simulink model "windEmulatorStep4"  (R2025b)
settings: Solver=ode4  StartTime=0.0  StopTime=inf  FixedStep=Ts  RelTol=1e-3
values from neighbouring files (symbols this model uses):
  A = 1.0    (= 1)    [initStep4.m]
  absEncoderCountsToRad = 1/2^20*2*pi    (= 5.99211245268e-06)    [initStep4.m]
  acs800CtrlStruct =     [windEmulatorBusDefs.mat]
  acs800DcBusVoltsScaling = 1    [initStep4.m]
  acs800FreqScaling = 1/100    (= 0.01)    [initStep4.m]
  acs800PowerScaling = Gen_PowerScaling    (= 14.9109)    [initStep4.m]
  acs800SignalStruct =     [windEmulatorBusDefs.mat]
  acs800SpeedNomEng = 1500    [initStep4.m]
  acs800SpeedNomFb = 20000    [initStep4.m]
  acs800SpeedScaling = 1500/20000    (= 0.075)    [initStep4.m]
  acs800TempScaling = 1/10    (= 0.1)    [initStep4.m]
  acs800TorqueNomEng = 100    [initStep4.m]
  acs800TorqueNomFb = 10000    [initStep4.m]
  acs800TorqueScaling = acs800TorqueRating/10000    (= 0.008035933)    [initStep4.m]
  acs880CtrlStruct =     [windEmulatorBusDefs.mat]
  acs880FreqScaling = 60/20000    (= 0.003)    [initStep4.m]
  acs880MotorCurrentScaling = 100/10000    (= 0.01)    [initStep4.m]
  acs880MotorVoltsScaling = 1    [initStep4.m]
  acs880PowerScaling = 100*hp2W/10000    (= 7.457)    [initStep4.m]
  acs880RatedTorque = 80.494    [initStep4.m]
  acs880RateLimFalling = -10000    [initStep4.m]
  acs880RateLimRising = 10000    [initStep4.m]
  acs880SetpointLimLower = -0.975*acs880RatedTorque    (= -78.48165)    [initStep4.m]
  acs880SetpointLimUpper = 0.975*acs880RatedTorque    (= 78.48165)    [initStep4.m]
  acs880SignalStruct =     [windEmulatorBusDefs.mat]
  acs880SpeedPILimLo = -0.975*acs880RatedTorque    (= -78.48165)    [initStep4.m]
  acs880SpeedPILimUp = 0.975*acs880RatedTorque    (= 78.48165)    [initStep4.m]
  acs880SpeedScaling = 2000/20000    (= 0.1)    [initStep4.m]
  acs880TorqueFieldbusScale = 10000    [initStep4.m]
  acs880TorqueScaling = acs880RatedTorque/acs880TorqueFieldbusScale    (= 0.0080494)    [initStep4.m]
  acs880TorqueSetpointScaling = 100    [initStep4.m]
  bar2pa = 1e5    (= 100000)    [initStep4.m]
  belowMinPGain = 1/200    (= 0.005)    [initStep4.m]
  ctrlModeTorque = logical(true)    [init.m]    (also in initStep1.m; initStep2.m; initStep3.m; initStep4.m)
  ctrlSignal1 = squeeze(hptoSignalsData.Values.ctrlSignal1.Data)    [postProcessingStep2.m]
  ctrlSignal2 = squeeze(hptoSignalsData.Values.ctrlSignal2.Data)    [postProcessingStep2.m]
  deadBandController = boolean(false)    [initStep4.m]
  deadbandTorqueSlewRate = 300    [initStep4.m]
  Dm_max = 40    [initStep4.m]
  EffMechMax = 0.93    [initStep4.m]
  EffMechMin = 0.79    [initStep4.m]
  excForce_N = squeeze(hptoCtrlData.Values.excForce_N.Data)    [postProcessingStep2.m]
  expCtrlStruct =     [windEmulatorBusDefs.mat]
  FactorEff = psi2pa*cc2m3*(1/rev2rad)    (= 0.00109733470463)    [initStep4.m]
  fromFileSpeedSlewRate = 250    [initStep4.m]
  fromFileTorqueSlewRate = 25    [initStep4.m]
  futekTorqueScale = -1/(2^31)*10/5*100    (= -9.31322574615e-08)    [initStep4.m]
  genMaxTorque = 0.8*ratedTorque    (= 64.3952)    [initStep3.m]    (also in initStep4.m = 78.48165)
  genTorqueCmd_Nm = squeeze(hptoSignalsData.Values.genTorqueCmd_Nm.Data)    [postProcessingStep2.m]
  hbmCtScale = 1/1.5    (= 0.666666666667)    [initStep4.m]
  hbmPowerStruct =     [windEmulatorBusDefs.mat]
  hptoCtrlStruct =     [windEmulatorBusDefs.mat]
  hptoSignalStruct =     [windEmulatorBusDefs.mat]
  invPowerStruct =     [windEmulatorBusDefs.mat]
  lpm2m3ps = 1/m3ps2lpm    (= 1.66666666667e-05)    [initStep4.m]
  minPressureRef_psi = 1000    [initStep4.m]
  minTorqueRef_Nm = (minPressureRef_psi*psi2pa)*(Dm_max*cc2m3*(1/rev2rad))    (= 43.8933881851)    [initStep4.m]
  motorSpeed_rpm = squeeze(acs880SignalsData.Values.motorSpeed_rpm.Data)    [postProcessingStep2.m]
  nPreDrop = 2900    [initStep4.m]
  nPreDropMin = 725    [initStep4.m]
  psi2bar = 1/bar2psi    (= 0.0689475729318)    [initStep4.m]
  radps2rpm = 60/(2*pi)    (= 9.54929658551)    [initStep2.m]    (also in initStep4.m)
  rpm2radps = 2*pi/60    (= 0.10471975512)    [initStep4.m]
  runCounter = squeeze(hptoCtrlData.Values.runCounter.Data)    [postProcessingStep2.m]
  shaftSignalStruct =     [windEmulatorBusDefs.mat]
  sidCtrlStruct =     [windEmulatorBusDefs.mat]
  sidDataCaseCounter = sidData.experimentData.count    [initStep4.m]
  sidDataSpeed_rpm = sidData.experimentData.wShaft_rpm    [initStep4.m]
  sidDataTorque_Nm = sidData.experimentData.torqueShaft_Nm    [initStep4.m]
  sidInfoStruct =     [windEmulatorBusDefs.mat]
  T = 4    [initStep4.m]
  targetOmega = 2000/60*2*pi    (= 209.439510239)    [initStep2.m]    (also in initStep3.m; initStep4.m)
  time = hptoCtrlData.Values.runCounter.Time    [postProcessingStep2.m]
  TorqueLoadMax = 75    [initStep4.m]
  Ts = 1/250    (= 0.004)    [initStep4.m]
undefined symbols (not defined in the file or in its folder): absEncoderCounts, absEncoderPosition_rad, absEncoderSpeed_rpm, absEncoderStatus1, absEncoderStatus2, absEncoderTurns, acs800Torque_Nm, acs800TorqueSetpoint_Nm, acs880SpeedSetpoint_rpm, acs880Torque_Nm, ctrlWord, dcBusVoltage_V, DiscIntNeverNeededParam, excShaftSpeed_rpm, excShaftTorque_Nm, expType, expTypeEnum, frequency_Hz, fromFileCaseCounter, genPumpFlow_lpm, genShaftSpeed_rpm, genSpeedActual, hmOutputShafTorque_Nm, motorCurrent_A, motorTorque_Nm, motorVoltage_V, pressure_bar, PressureControl, ramp, resetHilIntegrator, resetSidIntegrator, runHil, runSid, shaftPower_W, sidType, sidTypeEnum, SpeedControl, speedCtrlReset, speedRef_rpm, state, statusWord, stepCounter, temperature, torqueActual_Nm, TorqueInputControl, torqueSetpoint_Nm, torqueSetpoint_percent
libraries: slrealtimeethercatlib x118, fl_lib x26, nesl_utility x17, slrealtimeloglib x13, sh_lib x9, dspstat3 x5, simulink_extras x4, slpidlib x3, cstblocks x3, dspindex x3, simulink x2
(part 1 of 5)
settings Model: SimulationMode=external  Creator=SWEPT  LastModifiedBy=jleonqu
settings SolverCC: ConcurrentTasks=on  PositivePriorityOrder=on
settings DataIOCC: ExternalInput=inputData  LoadExternalInput=on
settings OptimizationCC: BlockReduction=off  OptimizeBlockIOStorage=off  ReuseModelBlockBuffer=off
settings DebuggingCC: TasksWithSamePriorityMsg=none  UnconnectedInputMsg=warning  UnconnectedOutputMsg=warning  UnconnectedLineMsg=warning
settings HardwareCC: ProdBitPerLong=64.0  ProdLongLongMode=on  ProdHWDeviceType=Intel->x86-64 (Linux 64)
settings ModelReferenceCC: EnableRefExpFcnMdlSchedulingChecks=on
settings RTWCC: SystemTargetFile=speedgoat.tlc  TemplateMakefile=slrealtime_default_tmf  RTWVerbose=off  Toolchain=Simulink Real-Time Toolchain  BuildConfiguration=Faster Runs  CodeExecutionProfiling=on  TargetLang=C++  GPUComputeCapability=3.5  DLArmComputeVersion=19.05  Description=Speedgoat Real-Time Target Machine
settings SimulinkRealTimeTargetCC: SLRTFileLogMaxRuns=1.0  ExtModeMaxTrigDuration=10.0  ExtModeStaticAllocSize=1000000.0  ExtModeTransport=0.0  MultiwordLength=2048.0  DynamicStringBufferSize=256.0  PreserveMATLABNamespacesInGeneratedCode=on  SubcomponentCodeInterfacePackaging=Reusable function  MATLABClassNameForMDSCustomization=Simulink.SoftwareTarget.GRTCustomization  InstructionSetFMA=off  LogToMDFFile=off

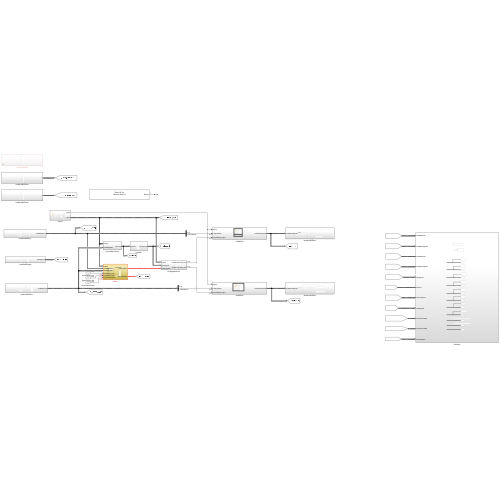
[thumbnail: Simulink's stored preview of the top-level diagram]
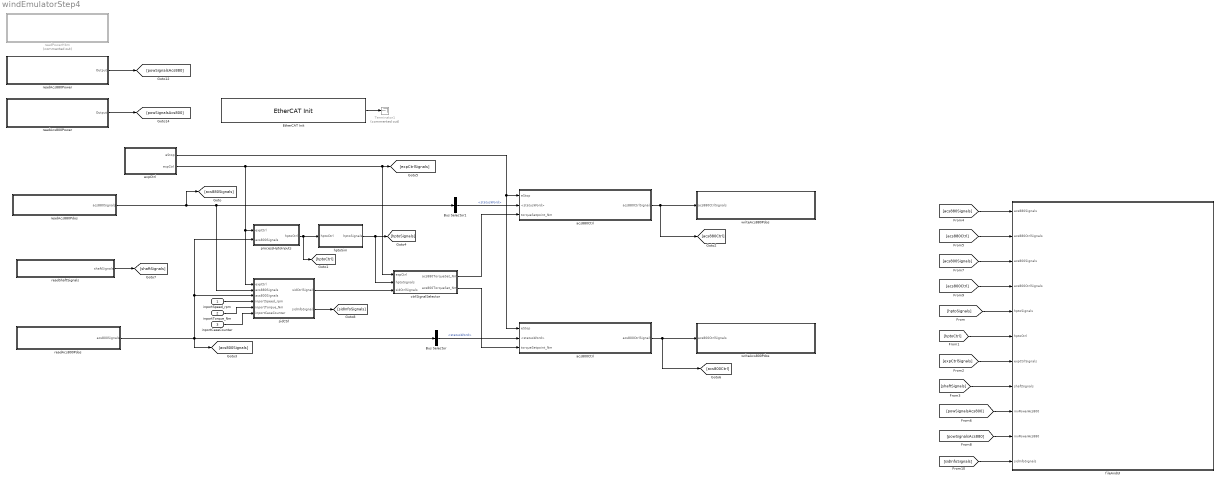
== system windEmulatorStep4 ==
  inportSpeed_rpm : Inport  Interpolate=off
  inportTorque_Nm : Inport  Port=2  Interpolate=off
  inportCaseCounter : Inport  Port=3  Interpolate=off
  Bus Selector : BusSelector  OutputSignals=statusWord
  Bus Selector1 : BusSelector  OutputSignals=statusWord
  EtherCAT Init : slrealtimeethercatlib/EtherCAT Init  Priority=0  config_file=C:\Users\jleonqu\Documents\GitHub\WEC-Sim_Applications\WEC-Sim_HIL\WindEmulatorFiles_edited\ethercat\newDevice3File_windEmulator_noHBM-2026-06-26.xml  device_id=0  portnum=1  initstate=2  dctuning=2  enaDebug=1  logFile='c:\dbglog.txt'  sample_time=0.004000  DCMode=0
  Terminator1 : Terminator  Commented=on
  acs800Ctrl : Subsystem
  acs880Ctrl : Subsystem
  ctrlSignalSelector : Subsystem
  expCtrl : Subsystem
  fileAndUI : Subsystem
  hptoSim : Subsystem
  processHptoInputs : Subsystem
  readAcs800Pdos : Subsystem
  readAcs800Power : Subsystem
  readAcs880Pdos : Subsystem
  readAcs880Power : Subsystem
  readPowerHbm : Subsystem  Commented=on
  readShaftSignals : Subsystem
  sidCtrl : Subsystem
  writeAcs800Pdos : Subsystem
  writeAcs880Pdos : Subsystem
  wires:
  EtherCAT Init/1 -> Terminator1/1
  readAcs800Pdos/1(acs800Signals) -> Bus Selector/1, [acs800Signals], processHptoInputs/2(acs800Signals), sidCtrl/3(acs800Signals)
  readAcs880Pdos/1(acs880Signals) -> sidCtrl/2(acs880Signals), Bus Selector1/1, [acs880Signals]
  Bus Selector1/1 -> acs880Ctrl/2(<statusWord>)  "<statusWord>"
  acs880Ctrl/1(acs880CtrlSignals) -> [acs880Ctrl], writeAcs880Pdos/1(acs880CtrlSignals)
  [acs880Signals] -> fileAndUI/1(acs880Signals)
  [acs880Ctrl] -> fileAndUI/2(acs880CtrlSignals)
  Bus Selector/1 -> acs800Ctrl/2(<statusWord>)  "<statusWord>"
  hptoSim/1(hptoSignals) -> ctrlSignalSelector/2(hptoSignals), [hptoSignals]
  expCtrl/1(eStop) -> acs800Ctrl/1(eStop), acs880Ctrl/1(eStop)
  acs800Ctrl/1(acs800CtrlSignals) -> [acs800Ctrl], writeAcs800Pdos/1(acs800CtrlSignals)
  [acs800Signals] -> fileAndUI/3(acs800Signals)
  [acs800Ctrl] -> fileAndUI/4(acs800CtrlSignals)
  processHptoInputs/1(hptoCtrl) -> [hptoCtrl], hptoSim/1(hptoCtrl)
  [hptoSignals] -> fileAndUI/5(hptoSignals)
  [hptoCtrl] -> fileAndUI/6(hptoCtrl)
  sidCtrl/1(sidCtrlSignals) -> ctrlSignalSelector/3(sidCtrlSignals)
  ctrlSignalSelector/1(acs880TorqueSet_Nm) -> acs880Ctrl/3(torqueSetpoint_Nm)
  ctrlSignalSelector/2(acs800TorqueSet_Nm) -> acs800Ctrl/3(torqueSetpoint_Nm)
  [expCtrlSignals] -> fileAndUI/7(expCtrlSignals)
  readShaftSignals/1(shaftSignals) -> [shaftSignals]
  [shaftSignals] -> fileAndUI/8(shaftSignals)
  expCtrl/2(expCtrl) -> ctrlSignalSelector/1(expCtrl), [expCtrlSignals], sidCtrl/1(expCtrl), processHptoInputs/1(expCtrl)
  readAcs800Power/1(Output) -> [powSignalsAcs800]
  readAcs880Power/1(Output) -> [powSignalsAcs880]
  [powSignalsAcs800] -> fileAndUI/9(invPowerAcs800)
  [powSignalsAcs880] -> fileAndUI/10(invPowerAcs880)
  sidCtrl/2(sidInfoSignals) -> [sidInfoSignals]
  [sidInfoSignals] -> fileAndUI/11(sidInfoSignals)
  inportSpeed_rpm/1 -> sidCtrl/4(inportSpeed_rpm)
  inportTorque_Nm/1 -> sidCtrl/5(inportTorque_Nm)
  inportCaseCounter/1 -> sidCtrl/6(inportCaseCounter)

== system windEmulatorStep4/acs800Ctrl ==
  note: Any limiting of the torque setpoint here?
  note: ideally change this; needs change to ctrlWord type
  note: ACS800 state control
  note: Act on change of button
  eStop : Inport  OutDataTypeStr=boolean
  <statusWord> : Inport  Port=2
  torqueSetpoint_Nm : Inport  Port=3
  ACS800CtrlMode : Constant  Value=ctrlModeTorque  OutDataTypeStr=boolean
  ACS880FieldbusControl : Subsystem
  Bus Assignment : BusAssignment  AssignedSignals=ctrlWord,state,torqueSetpoint_Nm,torqueSetpoint_percent
  Cast To Double : DataTypeConversion  OutDataTypeStr=double  SaturateOnIntegerOverflow=off  RndMeth=Floor
  Cast To Double1 : DataTypeConversion  OutDataTypeStr=int32  SaturateOnIntegerOverflow=off  RndMeth=Floor
  Constant : Constant  Value=acs800CtrlStruct  OutDataTypeStr=Bus: acs800CtrlBus
  Memory : Memory
  Memory1 : Memory
  Memory2 : Memory
  "Nm -> %" : Gain  Gain=1/acs880RatedTorque*100
  NotEqual : RelationalOperator  Operator=~=  OutDataTypeStr=boolean  RndMeth=Simplest  InputSameDT=off
  NotEqual1 : RelationalOperator  Operator=~=  OutDataTypeStr=boolean  RndMeth=Simplest  InputSameDT=off
  NotEqual2 : RelationalOperator  Operator=~=  OutDataTypeStr=boolean  RndMeth=Simplest  InputSameDT=off
  powerDownButton : Constant  Value=false
  powerUpButton : Constant  Value=false
  resetFaultButton : Constant  Value=false
  acs800CtrlSignals : Outport  OutDataTypeStr=Bus: acs800CtrlBus
  wires:
  <statusWord>/1 -> ACS880FieldbusControl/5(StatusWord)
  powerUpButton/1 -> NotEqual/1, Memory/1
  Memory/1 -> NotEqual/2
  ACS800CtrlMode/1 -> ACS880FieldbusControl/6(ctrlMode)
  Memory1/1 -> NotEqual1/2
  powerDownButton/1 -> NotEqual1/1, Memory1/1
  resetFaultButton/1 -> Memory2/1, NotEqual2/1
  Memory2/1 -> NotEqual2/2
  NotEqual/1 -> ACS880FieldbusControl/1(powerUp)
  NotEqual1/1 -> ACS880FieldbusControl/2(powerDown)
  eStop/1 -> ACS880FieldbusControl/4(eStop)
  ACS880FieldbusControl/2(state) -> Cast To Double1/1
  NotEqual2/1 -> Cast To Double/1
  Cast To Double/1 -> ACS880FieldbusControl/3(resetFault)
  Constant/1 -> Bus Assignment/1
  ACS880FieldbusControl/1(ControlWord) -> Bus Assignment/2
  Bus Assignment/1 -> acs800CtrlSignals/1
  Cast To Double1/1 -> Bus Assignment/3
  torqueSetpoint_Nm/1 -> Bus Assignment/4, "Nm -> %"/1
  "Nm -> %"/1 -> Bus Assignment/5

== system windEmulatorStep4/acs880Ctrl ==
  note: ideally change this; needs change to ctrlWord type
  note: ACS880 Control Word
  note: Act on change of button
  note: Should not need this ramp anymore; this was originally used for manual (constant) torque setpoints
  note: ACS880 Torque setpoint limit and conversion
  eStop : Inport  OutDataTypeStr=boolean
  <statusWord> : Inport  Port=2
  torqueSetpoint_Nm : Inport  Port=3  OutDataTypeStr=double
  ACS880CtrlMode : Constant  Value=ctrlModeTorque  OutDataTypeStr=boolean
  ACS880FieldbusControl : Subsystem
  ACS880Ramp : Stateflow chart  Commented=on  TreatAsAtomicUnit=on
  ACS880Setpoint : Product  Commented=on
  Bus Assignment : BusAssignment  AssignedSignals=ctrlWord,state,torqueSetpoint_Nm,torqueSetpoint_percent
  Cast To Double : DataTypeConversion  OutDataTypeStr=double  SaturateOnIntegerOverflow=off  RndMeth=Floor
  Cast To Double1 : DataTypeConversion  OutDataTypeStr=int32  SaturateOnIntegerOverflow=off  RndMeth=Floor
  Constant : Constant  Value=acs880CtrlStruct  OutDataTypeStr=Bus: acs880CtrlBus
  Memory : Memory
  Memory1 : Memory
  Memory2 : Memory
  "Nm -> %" : Gain  Gain=1/acs880RatedTorque*100
  NotEqual : RelationalOperator  Operator=~=  OutDataTypeStr=boolean  RndMeth=Simplest  InputSameDT=off
  NotEqual1 : RelationalOperator  Operator=~=  OutDataTypeStr=boolean  RndMeth=Simplest  InputSameDT=off
  NotEqual2 : RelationalOperator  Operator=~=  OutDataTypeStr=boolean  RndMeth=Simplest  InputSameDT=off
  Saturation : Saturate  UpperLimit=acs880SetpointLimUpper  LowerLimit=acs880SetpointLimLower
  acs880RateLim : RateLimiter  RisingSlewLimit=acs880RateLimRising  FallingSlewLimit=acs880RateLimFalling  SampleTimeMode=inherited
  powerDownButton : Constant  Value=false
  powerUpButton : Constant  Value=false
  resetFaultButton : Constant  Value=false
  acs880CtrlSignals : Outport  OutDataTypeStr=Bus: acs880CtrlBus
  wires:
  <statusWord>/1 -> ACS880FieldbusControl/5(StatusWord)
  powerUpButton/1 -> NotEqual/1, Memory/1
  Memory/1 -> NotEqual/2
  ACS880CtrlMode/1 -> ACS880FieldbusControl/6(ctrlMode)
  Memory1/1 -> NotEqual1/2
  powerDownButton/1 -> NotEqual1/1, Memory1/1
  resetFaultButton/1 -> Memory2/1, NotEqual2/1
  Memory2/1 -> NotEqual2/2
  NotEqual/1 -> ACS880FieldbusControl/1(powerUp)
  NotEqual1/1 -> ACS880FieldbusControl/2(powerDown)
  eStop/1 -> ACS880FieldbusControl/4(eStop)
  ACS880FieldbusControl/2(state) -> Cast To Double1/1
  NotEqual2/1 -> Cast To Double/1
  Cast To Double/1 -> ACS880FieldbusControl/3(resetFault)
  Constant/1 -> Bus Assignment/1
  ACS880FieldbusControl/1(ControlWord) -> Bus Assignment/2
  Bus Assignment/1 -> acs880CtrlSignals/1
  Cast To Double1/1 -> Bus Assignment/3
  ACS880Ramp/1(ramp) -> ACS880Setpoint/2  "rampValue"
  acs880RateLim/1 -> Saturation/1
  Saturation/1 -> "Nm -> %"/1, Bus Assignment/4  "ACS880Setpoint"
  torqueSetpoint_Nm/1 -> acs880RateLim/1
  "Nm -> %"/1 -> Bus Assignment/5

== system windEmulatorStep4/ctrlSignalSelector ==
  note: Modes:
      |
      | Off
      | Torque setpoint to both drives zero.
      |
      | SID
      | Torque setpoint to both drives taken from SID control signals.
      |
      | HIL
      | ACS880: simulates hydraulic machine (HM) output shaft
      | ACS800: provides the generator torque
  expCtrl : Inport  OutDataTypeStr=Bus: expCtrlBus
  hptoSignals : Inport  Port=2  OutDataTypeStr=Bus: hptoSignalBus
  sidCtrlSignals : Inport  Port=3  OutDataTypeStr=Bus: sidCtrlBus
  Bus Selector : BusSelector  OutputSignals=hmOutputShafTorque_Nm,genTorqueCmd_Nm
  Bus Selector1 : BusSelector  OutputSignals=acs880Torque_Nm,acs800Torque_Nm
  Bus Selector2 : BusSelector  OutputSignals=expType
  Multiport Switch : MultiPortSwitch  DataPortOrder=Specify indices  DataPortIndices={expTypeEnum.off,expTypeEnum.sid,expTypeEnum.hil}  DataPortForDefault=Additional data port  SaturateOnIntegerOverflow=off  InputSameDT=off
  Multiport Switch1 : MultiPortSwitch  DataPortOrder=Specify indices  DataPortIndices={expTypeEnum.off,expTypeEnum.sid,expTypeEnum.hil}  DataPortForDefault=Additional data port  SaturateOnIntegerOverflow=off  InputSameDT=off
  toExpTypeEnum : DataTypeConversion  OutDataTypeStr=Enum: expTypeEnum  SaturateOnIntegerOverflow=off  RndMeth=Floor
  zeroTorque : Constant  Value=0  OutDataTypeStr=double
  acs880TorqueSet_Nm : Outport
  acs800TorqueSet_Nm : Outport  Port=2
  wires:
  hptoSignals/1 -> Bus Selector/1
  sidCtrlSignals/1 -> Bus Selector1/1
  Multiport Switch/1 -> acs880TorqueSet_Nm/1
  Multiport Switch1/1 -> acs800TorqueSet_Nm/1
  zeroTorque/1 -> Multiport Switch1/5, Multiport Switch1/2, Multiport Switch/5, Multiport Switch/2
  Bus Selector1/1 -> Multiport Switch/3  "<acs880Torque_Nm>"
  Bus Selector1/2 -> Multiport Switch1/3  "<acs800Torque_Nm>"
  Bus Selector/1 -> Multiport Switch/4  "<hmOutputShafTorque_Nm>"
  Bus Selector/2 -> Multiport Switch1/4  "<genTorqueCmd_Nm>"
  Bus Selector2/1 -> toExpTypeEnum/1  "<expType>"
  expCtrl/1 -> Bus Selector2/1
  toExpTypeEnum/1 -> Multiport Switch1/1, Multiport Switch/1

== system windEmulatorStep4/expCtrl ==
  note: Act on change of button
  note: Act on change of button
  note: Act on change of button
  Bus Assignment : BusAssignment  AssignedSignals=expType,runHil,runSid,time,ramp,runCounter,stepCounter,resetHilIntegrator,resetSidIntegrator
  Constant : Constant  Value=expCtrlStruct  OutDataTypeStr=Bus: expCtrlBus
  Equal : RelationalOperator  Operator===  OutDataTypeStr=boolean  RndMeth=Simplest  InputSameDT=off
  Equal1 : RelationalOperator  Operator===  OutDataTypeStr=boolean  RndMeth=Simplest  InputSameDT=off
  FexcRamp : Stateflow chart  TreatAsAtomicUnit=on
  Memory : Memory
  Memory1 : Memory
  Memory2 : Memory
  NotEqual : RelationalOperator  Operator=~=  OutDataTypeStr=boolean  RndMeth=Simplest  InputSameDT=off
  NotEqual1 : RelationalOperator  Operator=~=  OutDataTypeStr=boolean  RndMeth=Simplest  InputSameDT=off
  NotEqual2 : RelationalOperator  Operator=~=  OutDataTypeStr=boolean  RndMeth=Simplest  InputSameDT=off
  ToUint16 : DataTypeConversion  OutDataTypeStr=uint16  SaturateOnIntegerOverflow=off  RndMeth=Floor
  eStopButton : Constant  Value=false
  expModeHil : Constant  Value=expTypeEnum.hil  OutDataTypeStr=Enum: expTypeEnum
  expModeSid : Constant  Value=expTypeEnum.sid  OutDataTypeStr=Enum: expTypeEnum
  expRunTime : Constant  Value=0
  expType : Constant  Value=expTypeEnum.off  OutDataTypeStr=Enum: expTypeEnum
  startButton : Constant  Value=false
  stopButton : Constant  Value=false
  eStop : Outport
  expCtrl : Outport  Port=2  OutDataTypeStr=Bus: expCtrlBus
  wires:
  eStopButton/1 -> NotEqual/1, Memory/1
  NotEqual/1 -> eStop/1
  Memory/1 -> NotEqual/2
  Bus Assignment/1 -> expCtrl/1
  Constant/1 -> Bus Assignment/1
  ToUint16/1 -> Bus Assignment/2
  expType/1 -> FexcRamp/1(expType), Equal1/1, Equal/1, ToUint16/1
  Memory1/1 -> NotEqual1/2
  startButton/1 -> Memory1/1, NotEqual1/1
  Memory2/1 -> NotEqual2/2
  stopButton/1 -> Memory2/1, NotEqual2/1
  NotEqual1/1 -> FexcRamp/2(startButton)
  NotEqual2/1 -> FexcRamp/3(stopButton)
  expRunTime/1 -> FexcRamp/4(expRunTime)
  FexcRamp/1(time) -> Bus Assignment/5
  FexcRamp/2(ramp) -> Bus Assignment/6  "rampValue"
  FexcRamp/3(runCounter) -> Bus Assignment/7
  Equal/1 -> Bus Assignment/3
  expModeHil/1 -> Equal/2
  Equal1/1 -> Bus Assignment/4
  expModeSid/1 -> Equal1/2
  FexcRamp/5(resetHilIntegrator) -> Bus Assignment/9
  FexcRamp/6(resetSidIntegrator) -> Bus Assignment/10
  FexcRamp/4(stepCounter) -> Bus Assignment/8

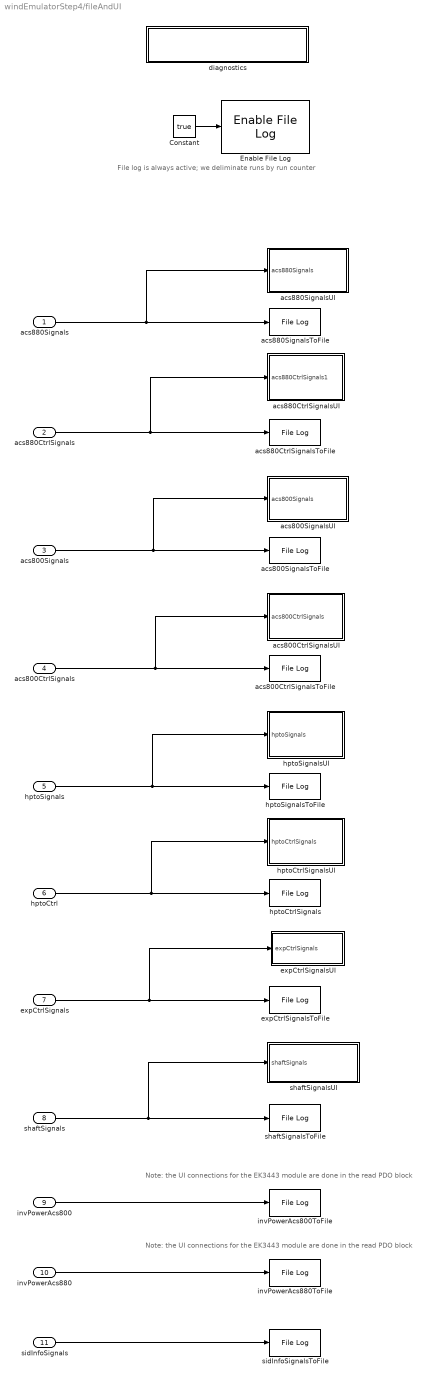
== system windEmulatorStep4/fileAndUI ==
  note: Note: the UI connections for the EK3443 module are done in the read PDO block
  note: File log is always active; we deliminate runs by run counter
  note: Note: the UI connections for the EK3443 module are done in the read PDO block
  acs880Signals : Inport  OutDataTypeStr=Bus: acs880SignalBus
  acs880CtrlSignals : Inport  Port=2  OutDataTypeStr=Bus: acs880CtrlBus
  acs800Signals : Inport  Port=3  OutDataTypeStr=Bus: acs800SignalBus
  acs800CtrlSignals : Inport  Port=4  OutDataTypeStr=Bus: acs800CtrlBus
  hptoSignals : Inport  Port=5  OutDataTypeStr=Bus: hptoSignalBus
  hptoCtrl : Inport  Port=6  OutDataTypeStr=Bus: hptoCtrlBus
  expCtrlSignals : Inport  Port=7  OutDataTypeStr=Bus: expCtrlBus
  shaftSignals : Inport  Port=8  OutDataTypeStr=Bus: shaftSignalBus
  invPowerAcs800 : Inport  Port=9  OutDataTypeStr=Bus: invPowerBus
  invPowerAcs880 : Inport  Port=10  OutDataTypeStr=Bus: invPowerBus
  sidInfoSignals : Inport  Port=11  OutDataTypeStr=Bus: sidInfoBus
  Constant : Constant  Value=true  OutDataTypeStr=boolean
  Enable File Log : slrealtimeloglib/Enable File Log
  acs800CtrlSignalsToFile : slrealtimeloglib/File Log  decimation=fileDecimation  inputProcessing=Elements as channels (sample based)
  acs800CtrlSignalsUI : Subsystem
  acs800SignalsToFile : slrealtimeloglib/File Log  decimation=fileDecimation  inputProcessing=Elements as channels (sample based)
  acs800SignalsUI : Subsystem
  acs880CtrlSignalsToFile : slrealtimeloglib/File Log  decimation=fileDecimation  inputProcessing=Elements as channels (sample based)
  acs880CtrlSignalsUI : Subsystem
  acs880SignalsToFile : slrealtimeloglib/File Log  decimation=fileDecimation  inputProcessing=Elements as channels (sample based)
  acs880SignalsUI : Subsystem
  diagnostics : Subsystem
  expCtrlSignalsToFile : slrealtimeloglib/File Log  decimation=fileDecimation  inputProcessing=Elements as channels (sample based)
  expCtrlSignalsUI : Subsystem
  hptoCtrlSignals : slrealtimeloglib/File Log  decimation=fileDecimation  inputProcessing=Elements as channels (sample based)
  hptoCtrlSignalsUI : Subsystem
  hptoSignalsToFile : slrealtimeloglib/File Log  decimation=fileDecimation  inputProcessing=Elements as channels (sample based)
  hptoSignalsUI : Subsystem
  invPowerAcs800ToFile : slrealtimeloglib/File Log  decimation=fileDecimation  inputProcessing=Elements as channels (sample based)
  invPowerAcs880ToFile : slrealtimeloglib/File Log  decimation=fileDecimation  inputProcessing=Elements as channels (sample based)
  shaftSignalsToFile : slrealtimeloglib/File Log  decimation=fileDecimation  inputProcessing=Elements as channels (sample based)
  shaftSignalsUI : Subsystem
  sidInfoSignalsToFile : slrealtimeloglib/File Log  decimation=fileDecimation  inputProcessing=Elements as channels (sample based)
  wires:
  Constant/1 -> Enable File Log/1
  acs880Signals/1 -> acs880SignalsUI/1(acs880Signals), acs880SignalsToFile/1
  acs880CtrlSignals/1 -> acs880CtrlSignalsUI/1(acs880CtrlSignals1), acs880CtrlSignalsToFile/1
  acs800Signals/1 -> acs800SignalsUI/1(acs800Signals), acs800SignalsToFile/1
  acs800CtrlSignals/1 -> acs800CtrlSignalsUI/1(acs800CtrlSignals), acs800CtrlSignalsToFile/1
  hptoSignals/1 -> hptoSignalsUI/1(hptoSignals), hptoSignalsToFile/1
  hptoCtrl/1 -> hptoCtrlSignalsUI/1(hptoCtrlSignals), hptoCtrlSignals/1
  expCtrlSignals/1 -> expCtrlSignalsUI/1(expCtrlSignals), expCtrlSignalsToFile/1
  shaftSignals/1 -> shaftSignalsToFile/1, shaftSignalsUI/1(shaftSignals)
  invPowerAcs800/1 -> invPowerAcs800ToFile/1
  invPowerAcs880/1 -> invPowerAcs880ToFile/1
  sidInfoSignals/1 -> sidInfoSignalsToFile/1

== system windEmulatorStep4/hptoSim ==
  note: Notes on Step 4:
      |
      | TODO: Review the below text; this is outdated.
      |
      | One drive is in torque control and the other is in speed control.
      |
      | The torque and shaft speed setpoint are produced as the output of the shaft in the hydraulic motor and generator in the hydraulic PTO model.
  hptoCtrl : Inport  OutDataTypeStr=Bus: hptoCtrlBus
  Bus Assignment : BusAssignment  AssignedSignals=genTorqueCmd_Nm,pressure_bar,hmOutputShafTorque_Nm,genShaftSpeed_rpm,excShaftSpeed_rpm,excShaftTorque_Nm,ctrlSignal1,ctrlSignal2,genPumpFlow_lpm
  Bus Selector : BusSelector  OutputSignals=speedRef_rpm,genSpeedActual,excForce_N,speedCtrlReset
  Constant : Constant  Value=hptoSignalStruct  OutDataTypeStr=Bus: hptoSignalBus
  hptoModel : Subsystem
  "psi -> bar" : Gain  Gain=psi2bar
  hptoSignals : Outport  OutDataTypeStr=Bus: hptoSignalBus
  wires:
  hptoModel/9(genPumpFlow_lpm) -> Bus Assignment/10
  hptoModel/3(hmOutputShaftTorque_Nm) -> Bus Assignment/4
  Bus Assignment/1 -> hptoSignals/1
  Constant/1 -> Bus Assignment/1
  hptoModel/4(genShaftSpeed_rpm) -> Bus Assignment/5
  hptoModel/8(controlSignal2) -> Bus Assignment/9
  hptoModel/1(genTorqueCmd_Nm) -> Bus Assignment/2  "genTorque_Nm"
  hptoModel/2(pressure_psi) -> "psi -> bar"/1  "pressure_psi"
  "psi -> bar"/1 -> Bus Assignment/3
  hptoModel/7(controlSignal1) -> Bus Assignment/8
  hptoCtrl/1 -> Bus Selector/1
  Bus Selector/1 -> hptoModel/1(speedReference)  "<speedRef_rpm>"
  Bus Selector/2 -> hptoModel/2(genSpeedActual_rpm)  "<genSpeedActual>"
  Bus Selector/3 -> hptoModel/3(excForce_N)  "<excForce_N>"
  Bus Selector/4 -> hptoModel/4(speedControllerReset)  "<speedCtrlReset>"
  hptoModel/5(excShaftSpeed_rpm) -> Bus Assignment/6
  hptoModel/6(excShaftTorque_Nm) -> Bus Assignment/7

== system windEmulatorStep4/processHptoInputs ==
  note: Keep exciation force at zero if we are not running HIL
  note: This is in (N) for the WaveBot excitation force
  expCtrl : Inport  OutDataTypeStr=Bus: expCtrlBus
  acs800Signals : Inport  Port=2  OutDataTypeStr=Bus: acs800SignalBus
  Bus Assignment : BusAssignment  AssignedSignals=speedRef_rpm,excForce_N,genSpeedActual,speedCtrlReset
  Bus Selector : BusSelector  OutputSignals=ramp,runHil,time,resetHilIntegrator
  Bus Selector2 : BusSelector  OutputSignals=motorSpeed_rpm
  Constant : Constant  Value=hptoCtrlStruct  OutDataTypeStr=Bus: hptoCtrlBus
  Constant1 : Constant  Value=0
  ExcitationForce_N : Product
  Product : Product
  Product4 : Product
  Rate Limiter : RateLimiter  RisingSlewLimit=50  FallingSlewLimit=-50  SampleTimeMode=inherited
  Sin2 : Trigonometry
  Switch : Switch  Criteria=u2 > Threshold  SaturateOnIntegerOverflow=off  InputSameDT=off
  excForceAmpNow_N : Gain
  excForceAmp_N : Constant  Value=0
  excForceFreq_Hz : Constant  Value=0
  f->w : Gain  Gain=2*pi
  speedReference : Constant  Value=0
  hptoCtrl : Outport  OutDataTypeStr=Bus: hptoCtrlBus
  wires:
  speedReference/1 -> Rate Limiter/1
  Rate Limiter/1 -> Bus Assignment/2
  Switch/1 -> Product/2  "rampValue"
  Product4/1 -> Sin2/1
  Sin2/1 -> ExcitationForce_N/1
  acs800Signals/1 -> Bus Selector2/1
  Constant/1 -> Bus Assignment/1
  Bus Assignment/1 -> hptoCtrl/1
  Bus Selector2/1 -> Bus Assignment/4  "<motorSpeed_rpm>"
  excForceFreq_Hz/1 -> f->w/1
  f->w/1 -> Product4/1
  ExcitationForce_N/1 -> Product/1  "waveBotExcitationForce_N"
  Product/1 -> Bus Assignment/3
  excForceAmp_N/1 -> excForceAmpNow_N/1
  excForceAmpNow_N/1 -> ExcitationForce_N/2
  expCtrl/1 -> Bus Selector/1
  Bus Selector/3 -> Product4/2  "<time>"
  Bus Selector/2 -> Switch/2  "<runHil>"
  Bus Selector/1 -> Switch/1  "<ramp>"
  Constant1/1 -> Switch/3
  Bus Selector/4 -> Bus Assignment/5  "<resetHilIntegrator>"

== system windEmulatorStep4/readAcs800Pdos ==
  Bus Assignment : BusAssignment  AssignedSignals=dcBusVoltage_V,frequency_Hz,temperature,motorSpeed_rpm,motorTorque_Nm,shaftPower_W,statusWord
  Constant : Constant  Value=acs800SignalStruct  OutDataTypeStr=Bus: acs800SignalBus
  Data Type Conversion{,1..5} (6 alike) : DataTypeConversion  OutDataTypeStr=double  SaturateOnIntegerOverflow=off  RndMeth=Floor
  EtherCAT PDO Receive10 : slrealtimeethercatlib/EtherCAT PDO Receive  Priority=2  sig_name=ACS800.TxPDO 1.Converter Temperature  sig_offset=632  sig_type=int16  type_size=16  sig_dim=1  device_id=0  sample_time=0.004000
  EtherCAT PDO Receive11 : slrealtimeethercatlib/EtherCAT PDO Receive  Priority=2  sig_name=ACS800.TxPDO 1.Actual Feedback (Transparent)  sig_offset=536  sig_type=int16  type_size=16  sig_dim=1  device_id=0  sample_time=0.004000
  EtherCAT PDO Receive12 : slrealtimeethercatlib/EtherCAT PDO Receive  Priority=2  sig_name=ACS800.TxPDO 1.Torque  sig_offset=568  sig_type=int16  type_size=16  sig_dim=1  device_id=0  sample_time=0.004000
  EtherCAT PDO Receive13 : slrealtimeethercatlib/EtherCAT PDO Receive  Priority=2  sig_name=ACS800.TxPDO 1.Power  sig_offset=584  sig_type=int16  type_size=16  sig_dim=1  device_id=0  sample_time=0.004000
  EtherCAT PDO Receive7 : slrealtimeethercatlib/EtherCAT PDO Receive  Priority=2  sig_name=ACS800.TxPDO 1.Main StatusWord (Transparent)  sig_offset=520  sig_type=uint16  type_size=16  sig_dim=1  device_id=0  sample_time=0.004000
  EtherCAT PDO Receive8 : slrealtimeethercatlib/EtherCAT PDO Receive  Priority=2  sig_name=ACS800.TxPDO 1.DC Bus Voltage  sig_offset=616  sig_type=int16  type_size=16  sig_dim=1  device_id=0  sample_time=0.004000
  EtherCAT PDO Receive9 : slrealtimeethercatlib/EtherCAT PDO Receive  Priority=2  sig_name=ACS800.TxPDO 1.Frequency  sig_offset=600  sig_type=int16  type_size=16  sig_dim=1  device_id=0  sample_time=0.004000
  Gain : Gain  Gain=acs800SpeedScaling
  Gain1 : Gain  Gain=acs800TorqueScaling
  Gain2 : Gain  Gain=acs800PowerScaling
  Gain3 : Gain  Gain=acs800DcBusVoltsScaling
  Gain4 : Gain  Gain=acs800FreqScaling
  Gain5 : Gain  Gain=acs800TempScaling
  acs800Signals : Outport  OutDataTypeStr=Bus: acs800SignalBus
  wires:
  Data Type Conversion/1 -> Gain/1
  EtherCAT PDO Receive11/1 -> Data Type Conversion/1  "ACS800ActualFeedback"
  Constant/1 -> Bus Assignment/1
  EtherCAT PDO Receive12/1 -> Data Type Conversion1/1  "ACS800Torque"
  Data Type Conversion1/1 -> Gain1/1
  EtherCAT PDO Receive13/1 -> Data Type Conversion2/1  "ACS800Power"
  Data Type Conversion2/1 -> Gain2/1
  Gain2/1 -> Bus Assignment/7
  Bus Assignment/1 -> acs800Signals/1
  EtherCAT PDO Receive9/1 -> Data Type Conversion3/1  "ACS800Frequency"
  EtherCAT PDO Receive8/1 -> Data Type Conversion4/1  "ACS800DcBusVoltage"
  EtherCAT PDO Receive10/1 -> Data Type Conversion5/1  "ACS800Temperature"
  Data Type Conversion4/1 -> Gain3/1
  Gain3/1 -> Bus Assignment/2
  Data Type Conversion3/1 -> Gain4/1
  Data Type Conversion5/1 -> Gain5/1
  Gain4/1 -> Bus Assignment/3
  Gain5/1 -> Bus Assignment/4
  EtherCAT PDO Receive7/1 -> Bus Assignment/8  "ACS800StatusWord"
  Gain1/1 -> Bus Assignment/6
  Gain/1 -> Bus Assignment/5

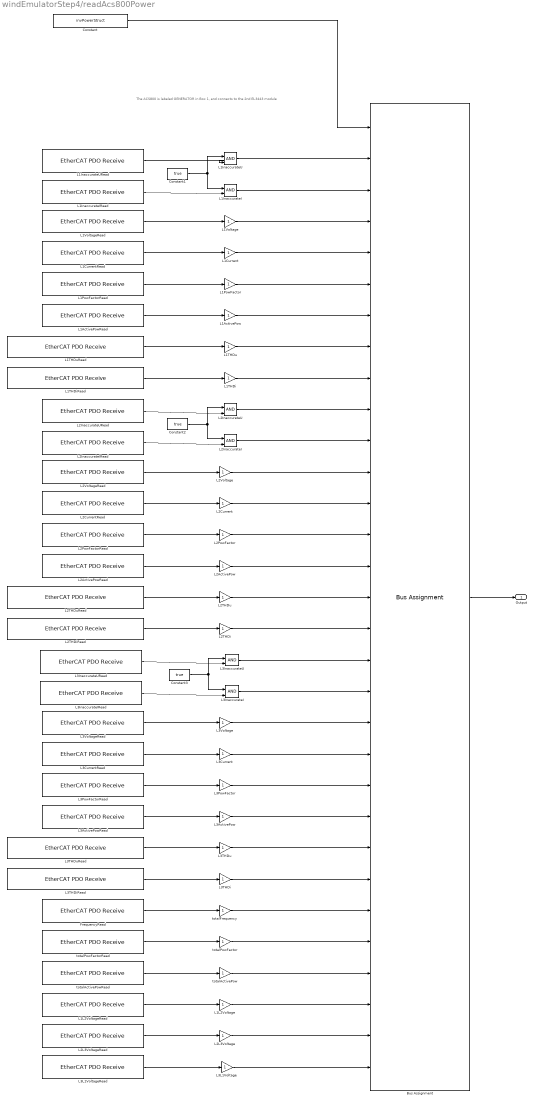
== system windEmulatorStep4/readAcs800Power ==
  note: The ACS800 is labeled GENERATOR in Box 1, and connects to the 2nd EL3443 module
  Bus Assignment : BusAssignment  AssignedSignals=L1InaccurateU,L1InaccurateI,L1Voltage,L1Current,L1PowFactor,L1ActivePow,L1THDu,L1THDi,L2InaccurateU,L2InaccurateI,L2Voltage,L2Current,L2PowFactor,L2ActivePow,L2THDu,L2THDi,L3InaccurateU,L3InaccurateI,L3Voltage,L3Current,L3PowFactor,L3ActivePow,L3THDu,L3THDi,Frequency,TotalPowFactor,TotalActivePow,L1L2Voltage,L2L3Voltage,L3L1Volage
  Constant : Constant  Value=invPowerStruct  OutDataTypeStr=Bus: invPowerBus
  Constant1 : Constant  Value=true  OutDataTypeStr=boolean
  Constant2 : Constant  Value=true  OutDataTypeStr=boolean
  Constant3 : Constant  Value=true  OutDataTypeStr=boolean
  FrequencyRead : slrealtimeethercatlib/EtherCAT PDO Receive  Priority=2  sig_name=POW_EL3443_02.Total Basic.Frequency  sig_offset=3992  sig_type=single  type_size=32  sig_dim=1  device_id=0  sample_time=0.004000
  L1ActivePow : Gain  OutDataTypeStr=double
  L1ActivePowRead : slrealtimeethercatlib/EtherCAT PDO Receive  Priority=2  sig_name=POW_EL3443_02.L1 Power.Active Power  sig_offset=2776  sig_type=single  type_size=32  sig_dim=1  device_id=0  sample_time=0.004000
  L1Current : Gain  OutDataTypeStr=double
  L1CurrentRead : slrealtimeethercatlib/EtherCAT PDO Receive  Priority=2  sig_name=POW_EL3443_02.L1 Basic.Current  sig_offset=2744  sig_type=single  type_size=32  sig_dim=1  device_id=0  sample_time=0.004000
  L1InaccurateI : Logic  IconShape=distinctive  AllPortsSameDT=off  OutDataTypeStr=boolean
  L1InaccurateIRead : slrealtimeethercatlib/EtherCAT PDO Receive  Priority=2  sig_name=POW_EL3443_02.L1 Status.Inaccurate Current  sig_offset=2700  sig_type=boolean  type_size=1  sig_dim=1  device_id=0  sample_time=0.004000
  L1InaccurateU : Logic  IconShape=distinctive  AllPortsSameDT=off  OutDataTypeStr=boolean
  L1InaccurateURead : slrealtimeethercatlib/EtherCAT PDO Receive  Priority=2  sig_name=POW_EL3443_02.L1 Status.Inaccurate Voltage  sig_offset=2699  sig_type=boolean  type_size=1  sig_dim=1  device_id=0  sample_time=0.004000
  L1L2Voltage : Gain  OutDataTypeStr=double
  L1L2VoltageRead : slrealtimeethercatlib/EtherCAT PDO Receive  Priority=2  sig_name=POW_EL3443_02.Total L-L Voltage.L1-L2 Voltage  sig_offset=4312  sig_type=single  type_size=32  sig_dim=1  device_id=0  sample_time=0.004000
  L1PowFactor : Gain  OutDataTypeStr=double
  L1PowFactorRead : slrealtimeethercatlib/EtherCAT PDO Receive  Priority=2  sig_name=POW_EL3443_02.L1 Power.Power Factor  sig_offset=2872  sig_type=single  type_size=32  sig_dim=1  device_id=0  sample_time=0.004000
  L1THDi : Gain  OutDataTypeStr=double
  L1THDiRead : slrealtimeethercatlib/EtherCAT PDO Receive  Priority=2  sig_name=POW_EL3443_02.L1 Advanced.Current Total Harmonic Distortion  sig_offset=3048  sig_type=single  type_size=32  sig_dim=1  device_id=0  sample_time=0.004000
  L1THDu : Gain  OutDataTypeStr=double
  L1THDuRead : slrealtimeethercatlib/EtherCAT PDO Receive  Priority=2  sig_name=POW_EL3443_02.L1 Advanced.Voltage Total Harmonic Distortion  sig_offset=2984  sig_type=single  type_size=32  sig_dim=1  device_id=0  sample_time=0.004000
  L1Voltage : Gain  OutDataTypeStr=double
  L1VoltageRead : slrealtimeethercatlib/EtherCAT PDO Receive  Priority=2  sig_name=POW_EL3443_02.L1 Basic.Voltage  sig_offset=2712  sig_type=single  type_size=32  sig_dim=1  device_id=0  sample_time=0.004000
  L2ActivePow : Gain  OutDataTypeStr=double
  L2ActivePowRead : slrealtimeethercatlib/EtherCAT PDO Receive  Priority=2  sig_name=POW_EL3443_02.L2 Power.Active Power  sig_offset=3192  sig_type=single  type_size=32  sig_dim=1  device_id=0  sample_time=0.004000
  L2Current : Gain  OutDataTypeStr=double
  L2CurrentRead : slrealtimeethercatlib/EtherCAT PDO Receive  Priority=2  sig_name=POW_EL3443_02.L2 Basic.Current  sig_offset=3160  sig_type=single  type_size=32  sig_dim=1  device_id=0  sample_time=0.004000
  L2InaccurateI : Logic  IconShape=distinctive  AllPortsSameDT=off  OutDataTypeStr=boolean
  L2InaccurateIRead : slrealtimeethercatlib/EtherCAT PDO Receive  Priority=2  sig_name=POW_EL3443_02.L2 Status.Inaccurate Current  sig_offset=3116  sig_type=boolean  type_size=1  sig_dim=1  device_id=0  sample_time=0.004000
  L2InaccurateU : Logic  IconShape=distinctive  AllPortsSameDT=off  OutDataTypeStr=boolean
  L2InaccurateURead : slrealtimeethercatlib/EtherCAT PDO Receive  Priority=2  sig_name=POW_EL3443_02.L2 Status.Inaccurate Voltage  sig_offset=3115  sig_type=boolean  type_size=1  sig_dim=1  device_id=0  sample_time=0.004000
  L2L3Voltage : Gain  OutDataTypeStr=double
  L2L3VoltageRead : slrealtimeethercatlib/EtherCAT PDO Receive  Priority=2  sig_name=POW_EL3443_02.Total L-L Voltage.L2-L3 Voltage  sig_offset=4344  sig_type=single  type_size=32  sig_dim=1  device_id=0  sample_time=0.004000
  L2PowFactor : Gain  OutDataTypeStr=double
  L2PowFactorRead : slrealtimeethercatlib/EtherCAT PDO Receive  Priority=2  sig_name=POW_EL3443_02.L2 Power.Power Factor  sig_offset=3288  sig_type=single  type_size=32  sig_dim=1  device_id=0  sample_time=0.004000
  L2THDi : Gain  OutDataTypeStr=double
  L2THDiRead : slrealtimeethercatlib/EtherCAT PDO Receive  Priority=2  sig_name=POW_EL3443_02.L2 Advanced.Current Total Harmonic Distortion  sig_offset=3464  sig_type=single  type_size=32  sig_dim=1  device_id=0  sample_time=0.004000
  L2THDu : Gain  OutDataTypeStr=double
  L2THDuRead : slrealtimeethercatlib/EtherCAT PDO Receive  Priority=2  sig_name=POW_EL3443_02.L2 Advanced.Voltage Total Harmonic Distortion  sig_offset=3400  sig_type=single  type_size=32  sig_dim=1  device_id=0  sample_time=0.004000
  L2Voltage : Gain  OutDataTypeStr=double
  L2VoltageRead : slrealtimeethercatlib/EtherCAT PDO Receive  Priority=2  sig_name=POW_EL3443_02.L2 Basic.Voltage  sig_offset=3128  sig_type=single  type_size=32  sig_dim=1  device_id=0  sample_time=0.004000
  L3ActivePow : Gain  OutDataTypeStr=double
  L3ActivePowRead : slrealtimeethercatlib/EtherCAT PDO Receive  Priority=2  sig_name=POW_EL3443_02.L3 Power.Active Power  sig_offset=3608  sig_type=single  type_size=32  sig_dim=1  device_id=0  sample_time=0.004000
  L3Current : Gain  OutDataTypeStr=double
  L3CurrentRead : slrealtimeethercatlib/EtherCAT PDO Receive  Priority=2  sig_name=POW_EL3443_02.L3 Basic.Current  sig_offset=3576  sig_type=single  type_size=32  sig_dim=1  device_id=0  sample_time=0.004000
  L3InaccurateI : Logic  IconShape=distinctive  AllPortsSameDT=off  OutDataTypeStr=boolean
  L3InaccurateIRead : slrealtimeethercatlib/EtherCAT PDO Receive  Priority=2  sig_name=POW_EL3443_02.L3 Status.Inaccurate Current  sig_offset=3532  sig_type=boolean  type_size=1  sig_dim=1  device_id=0  sample_time=0.004000
  L3InaccurateU : Logic  IconShape=distinctive  AllPortsSameDT=off  OutDataTypeStr=boolean
  L3InaccurateURead : slrealtimeethercatlib/EtherCAT PDO Receive  Priority=2  sig_name=POW_EL3443_02.L3 Status.Inaccurate Voltage  sig_offset=3531  sig_type=boolean  type_size=1  sig_dim=1  device_id=0  sample_time=0.004000
  L3L1Voltage : Gain  OutDataTypeStr=double
  L3L1VoltageRead : slrealtimeethercatlib/EtherCAT PDO Receive  Priority=2  sig_name=POW_EL3443_02.Total L-L Voltage.L3-L1 Voltage  sig_offset=4376  sig_type=single  type_size=32  sig_dim=1  device_id=0  sample_time=0.004000
  L3PowFactor : Gain  OutDataTypeStr=double
  L3PowFactorRead : slrealtimeethercatlib/EtherCAT PDO Receive  Priority=2  sig_name=POW_EL3443_02.L3 Power.Power Factor  sig_offset=3704  sig_type=single  type_size=32  sig_dim=1  device_id=0  sample_time=0.004000
  L3THDi : Gain  OutDataTypeStr=double
  L3THDiRead : slrealtimeethercatlib/EtherCAT PDO Receive  Priority=2  sig_name=POW_EL3443_02.L3 Advanced.Current Total Harmonic Distortion  sig_offset=3880  sig_type=single  type_size=32  sig_dim=1  device_id=0  sample_time=0.004000
  L3THDu : Gain  OutDataTypeStr=double
  L3THDuRead : slrealtimeethercatlib/EtherCAT PDO Receive  Priority=2  sig_name=POW_EL3443_02.L3 Advanced.Voltage Total Harmonic Distortion  sig_offset=3816  sig_type=single  type_size=32  sig_dim=1  device_id=0  sample_time=0.004000
  L3Voltage : Gain  OutDataTypeStr=double
  L3VoltageRead : slrealtimeethercatlib/EtherCAT PDO Receive  Priority=2  sig_name=POW_EL3443_02.L3 Basic.Voltage  sig_offset=3544  sig_type=single  type_size=32  sig_dim=1  device_id=0  sample_time=0.004000
  totalActivePow : Gain  OutDataTypeStr=double
  totalActivePowRead : slrealtimeethercatlib/EtherCAT PDO Receive  Priority=2  sig_name=POW_EL3443_02.Total Active.Active Power  sig_offset=4088  sig_type=single  type_size=32  sig_dim=1  device_id=0  sample_time=0.004000
  totalFrequency : Gain  OutDataTypeStr=double
  totalPowFactor : Gain  OutDataTypeStr=double
  totalPowFactorRead : slrealtimeethercatlib/EtherCAT PDO Receive  Priority=2  sig_name=POW_EL3443_02.Total Basic.Power Factor  sig_offset=4024  sig_type=single  type_size=32  sig_dim=1  device_id=0  sample_time=0.004000
  Output : Outport  OutDataTypeStr=Bus: invPowerBus
  wires:
  L3L1Voltage/1 -> Bus Assignment/31
  L3L1VoltageRead/1 -> L3L1Voltage/1
  L2L3VoltageRead/1 -> L2L3Voltage/1
  L2L3Voltage/1 -> Bus Assignment/30
  L1L2Voltage/1 -> Bus Assignment/29
  L1L2VoltageRead/1 -> L1L2Voltage/1
  totalActivePow/1 -> Bus Assignment/28
  totalActivePowRead/1 -> totalActivePow/1
  totalPowFactor/1 -> Bus Assignment/27
  totalPowFactorRead/1 -> totalPowFactor/1
  totalFrequency/1 -> Bus Assignment/26
  FrequencyRead/1 -> totalFrequency/1
  L3InaccurateURead/1 -> L3InaccurateU/2
  Constant3/1 -> L3InaccurateI/1, L3InaccurateU/1
  L3InaccurateIRead/1 -> L3InaccurateI/2
  L3InaccurateI/1 -> Bus Assignment/19
  L3InaccurateU/1 -> Bus Assignment/18
  L2InaccurateU/1 -> Bus Assignment/10
  L2InaccurateIRead/1 -> L2InaccurateI/2
  L2InaccurateI/1 -> Bus Assignment/11
  L2InaccurateURead/1 -> L2InaccurateU/2
  Constant2/1 -> L2InaccurateI/1, L2InaccurateU/1
  L1InaccurateIRead/1 -> L1InaccurateI/2
  L1InaccurateI/1 -> Bus Assignment/3
  L1InaccurateURead/1 -> L1InaccurateU/2
  L1InaccurateU/1 -> Bus Assignment/2
  Constant1/1 -> L1InaccurateI/1, L1InaccurateU/1
  L3THDiRead/1 -> L3THDi/1
  L3THDi/1 -> Bus Assignment/25
  L3THDu/1 -> Bus Assignment/24
  L3THDuRead/1 -> L3THDu/1
  L3ActivePow/1 -> Bus Assignment/23
  L3ActivePowRead/1 -> L3ActivePow/1
  L3PowFactor/1 -> Bus Assignment/22
  L3PowFactorRead/1 -> L3PowFactor/1
  L3Current/1 -> Bus Assignment/21
  L3CurrentRead/1 -> L3Current/1
  L3Voltage/1 -> Bus Assignment/20
  L3VoltageRead/1 -> L3Voltage/1
  L2VoltageRead/1 -> L2Voltage/1
  L2Voltage/1 -> Bus Assignment/12
  L2CurrentRead/1 -> L2Current/1
  L2Current/1 -> Bus Assignment/13
  L2PowFactorRead/1 -> L2PowFactor/1
  L2PowFactor/1 -> Bus Assignment/14
  L2ActivePowRead/1 -> L2ActivePow/1
  L2ActivePow/1 -> Bus Assignment/15
  L2THDuRead/1 -> L2THDu/1
  L2THDu/1 -> Bus Assignment/16
  L2THDi/1 -> Bus Assignment/17
  L2THDiRead/1 -> L2THDi/1
  L1THDiRead/1 -> L1THDi/1
  L1THDi/1 -> Bus Assignment/9
  L1THDu/1 -> Bus Assignment/8
  L1THDuRead/1 -> L1THDu/1
  L1ActivePow/1 -> Bus Assignment/7
  L1ActivePowRead/1 -> L1ActivePow/1
  L1PowFactor/1 -> Bus Assignment/6
  L1PowFactorRead/1 -> L1PowFactor/1
  L1Current/1 -> Bus Assignment/5
  L1CurrentRead/1 -> L1Current/1
  L1Voltage/1 -> Bus Assignment/4
  Bus Assignment/1 -> Output/1
  Constant/1 -> Bus Assignment/1
  L1VoltageRead/1 -> L1Voltage/1

== system windEmulatorStep4/readAcs880Pdos ==
  Bus Assignment : BusAssignment  AssignedSignals=motorVoltage_V,motorCurrent_A,frequency_Hz,motorSpeed_rpm,motorTorque_Nm,shaftPower_W,statusWord
  Cast To Double{,1..3} (4 alike) : DataTypeConversion  OutDataTypeStr=double  SaturateOnIntegerOverflow=off  RndMeth=Floor
  Constant : Constant  Value=acs880SignalStruct  OutDataTypeStr=Bus: acs880SignalBus
  Data Type Conversion1 : DataTypeConversion  OutDataTypeStr=double  SaturateOnIntegerOverflow=off  RndMeth=Floor
  Data Type Conversion2 : DataTypeConversion  OutDataTypeStr=double  SaturateOnIntegerOverflow=off  RndMeth=Floor
  EtherCAT PDO Receive : slrealtimeethercatlib/EtherCAT PDO Receive  Priority=2  sig_name=ACS880.TxPDO 1.ABB Drives Status Word  sig_offset=344  sig_type=uint16  type_size=16  sig_dim=1  device_id=0  sample_time=0.004000
  EtherCAT PDO Receive1 : slrealtimeethercatlib/EtherCAT PDO Receive  Priority=2  sig_name=ACS880.TxPDO 6.Calculated motor voltage  sig_offset=440  sig_type=int16  type_size=16  sig_dim=1  device_id=0  sample_time=0.004000
  EtherCAT PDO Receive2 : slrealtimeethercatlib/EtherCAT PDO Receive  Priority=2  sig_name=ACS880.TxPDO 6.Measured motor current  sig_offset=424  sig_type=int16  type_size=16  sig_dim=1  device_id=0  sample_time=0.004000
  EtherCAT PDO Receive3 : slrealtimeethercatlib/EtherCAT PDO Receive  Priority=2  sig_name=ACS880.TxPDO 6.Estimated output frequency  sig_offset=408  sig_type=int16  type_size=16  sig_dim=1  device_id=0  sample_time=0.004000
  EtherCAT PDO Receive4 : slrealtimeethercatlib/EtherCAT PDO Receive  Priority=2  sig_name=ACS880.TxPDO 6.Motor speed used  sig_offset=392  sig_type=int16  type_size=16  sig_dim=1  device_id=0  sample_time=0.004000
  EtherCAT PDO Receive5 : slrealtimeethercatlib/EtherCAT PDO Receive  Priority=2  sig_name=ACS880.TxPDO 6.Motor torque  sig_offset=456  sig_type=int16  type_size=16  sig_dim=1  device_id=0  sample_time=0.004000
  EtherCAT PDO Receive6 : slrealtimeethercatlib/EtherCAT PDO Receive  Priority=2  sig_name=ACS880.TxPDO 6.Estimated motor shaft power  sig_offset=472  sig_type=int16  type_size=16  sig_dim=1  device_id=0  sample_time=0.004000
  Gain : Gain  Gain=acs880MotorVoltsScaling
  Gain1 : Gain  Gain=acs880TorqueScaling
  Gain2 : Gain  Gain=acs880MotorCurrentScaling
  Gain3 : Gain  Gain=acs880FreqScaling
  Gain4 : Gain  Gain=acs880SpeedScaling
  Gain5 : Gain  Gain=acs880PowerScaling
  acs880Signals : Outport  OutDataTypeStr=Bus: acs880SignalBus
  wires:
  Data Type Conversion1/1 -> Gain1/1
  EtherCAT PDO Receive5/1 -> Data Type Conversion1/1  "ACS880MotorTorque"
  Constant/1 -> Bus Assignment/1
  Cast To Double/1 -> Gain/1
  EtherCAT PDO Receive1/1 -> Cast To Double/1  "ACS880MotorVoltage"
  Gain/1 -> Bus Assignment/2
  EtherCAT PDO Receive2/1 -> Cast To Double1/1  "ACS880MotorCurrent"
  Cast To Double1/1 -> Gain2/1
  Gain2/1 -> Bus Assignment/3
  EtherCAT PDO Receive3/1 -> Cast To Double2/1  "ACS880OutputFreq"
  Cast To Double2/1 -> Gain3/1
  Gain3/1 -> Bus Assignment/4
  EtherCAT PDO Receive4/1 -> Cast To Double3/1  "ACS880MotorSpeed"
  Cast To Double3/1 -> Gain4/1
  Gain4/1 -> Bus Assignment/5
  EtherCAT PDO Receive6/1 -> Data Type Conversion2/1  "ACS880MotorShaftPower"
  Data Type Conversion2/1 -> Gain5/1
  Gain5/1 -> Bus Assignment/7
  Bus Assignment/1 -> acs880Signals/1
  EtherCAT PDO Receive/1 -> Bus Assignment/8
  Gain1/1 -> Bus Assignment/6
